simulink model "trojpolozeniowy"  (R2023b)
settings: Solver=ode1  StartTime=0.0  StopTime=20  FixedStep=0.01  RelTol=1e-3
undefined symbols (not defined in the file): eps1, eps2
settings Model: Creator=Paweł  LastModifiedBy=Paweł

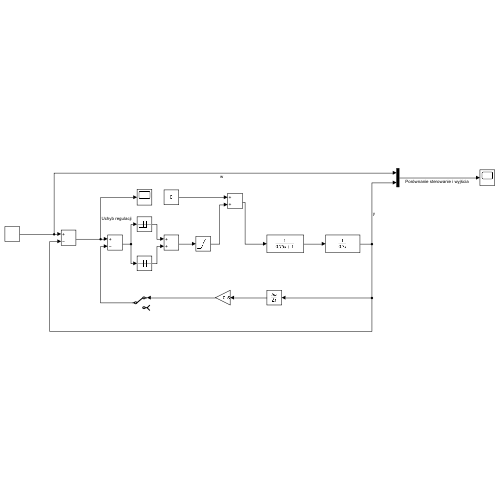
[thumbnail: Simulink's stored preview of the top-level diagram]
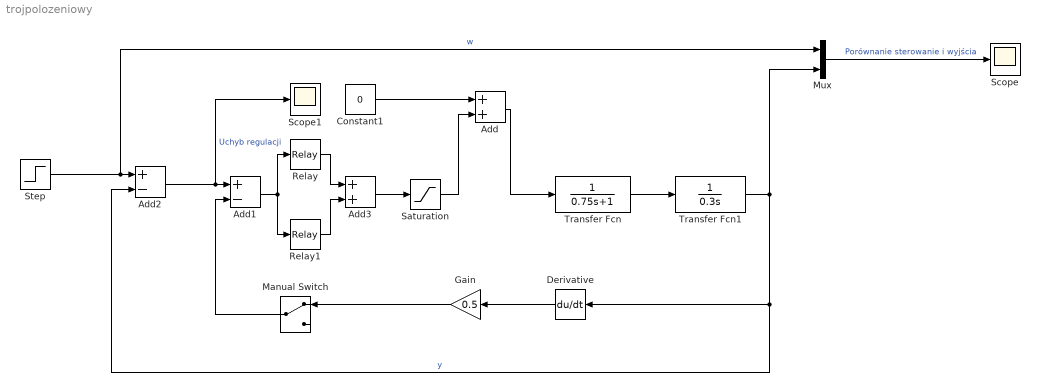
== system trojpolozeniowy ==
  Add : Sum
  Add1 : Sum  Inputs=+-
  Add2 : Sum  Inputs=+-
  Add3 : Sum
  Constant1 : Constant  Value=0
  Derivative : Derivative
  Gain : Gain  Gain=0.5
  Manual Switch : ManualSwitch
  Mux : Mux  Inputs=2
  Relay : Relay  OnSwitchValue=eps2  OffSwitchValue=eps1  OnOutputValue=5
  Relay1 : Relay  OnSwitchValue=-eps1  OffSwitchValue=-eps2  OnOutputValue=0  OffOutputValue=-5
  Saturation : Saturate  UpperLimit=5  LowerLimit=-5
  Scope : Scope
  Scope1 : Scope
  Step : Step  After=2  SampleTime=0
  Transfer Fcn : TransferFcn  Denominator=[0.75 1]
  Transfer Fcn1 : TransferFcn  Denominator=[0.3 0]
  wires:
  Step/1 -> Mux/1, Add2/1  "w"
  Manual Switch/1 -> Add1/2
  Derivative/1 -> Gain/1
  Gain/1 -> Manual Switch/1
  Transfer Fcn1/1 -> Mux/2, Derivative/1, Add2/2  "y"
  Add/1 -> Transfer Fcn/1
  Transfer Fcn/1 -> Transfer Fcn1/1
  Mux/1 -> Scope/1  "Porównanie sterowanie i wyjścia"
  Saturation/1 -> Add/2
  Constant1/1 -> Add/1
  Add2/1 -> Scope1/1, Add1/1  "Uchyb regulacji"
  Add3/1 -> Saturation/1
  Add1/1 -> Relay/1, Relay1/1
  Relay1/1 -> Add3/2
  Relay/1 -> Add3/1
